simulink subsystem "BS"  (R2024a)
settings: Solver=VariableStepAuto  StartTime=0.0  StopTime=10.0  RelTol=1e-3
settings Model: Creator=mrvol  LastModifiedBy=mrvol

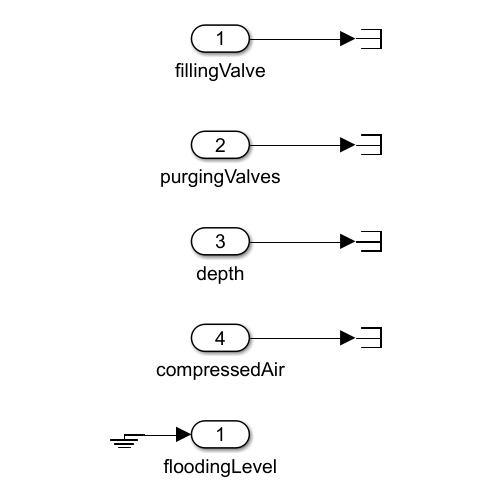
[thumbnail: Simulink's stored preview of the top-level diagram]
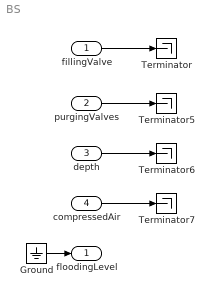
== system BS ==
  fillingValve : Inport
  purgingValves : Inport  Port=2
  depth : Inport  Port=3
  compressedAir : Inport  Port=4
  Ground : Ground
  Terminator{,5..7} (4 alike) : Terminator
  floodingLevel : Outport
  wires:
  Ground/1 -> floodingLevel/1
  fillingValve/1 -> Terminator/1
  purgingValves/1 -> Terminator5/1
  depth/1 -> Terminator6/1
  compressedAir/1 -> Terminator7/1
